simulink model "Batter_Model_01"  (R2013a)
settings: Solver=ode45  StartTime=0.0  StopTime=10.0  RelTol=1e-3
settings Model: Creator=hlopez5  LastModifiedBy=hlopez5

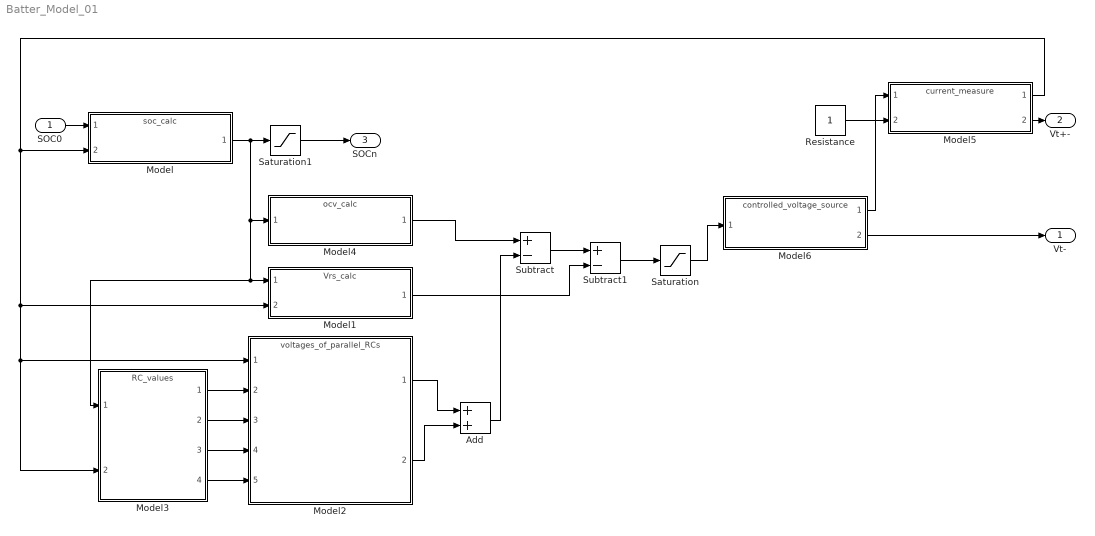
== system Batter_Model_01 ==
  SOC0 : Inport
  Add : Sum
  Model : ModelReference  ModelNameDialog=soc_calc.mdl  SimulationMode=Normal  ModelReferenceVersion=1.1  CopyOfModelName=soc_calc.mdl  DefaultDataLogging=on
  Model1 : ModelReference  ModelNameDialog=Vrs_calc.mdl  SimulationMode=Normal  ModelReferenceVersion=1.1  CopyOfModelName=Vrs_calc.mdl  DefaultDataLogging=on
  Model2 : ModelReference  ModelNameDialog=voltages_of_parallel_RCs.mdl  SimulationMode=Normal  ModelReferenceVersion=1.3  CopyOfModelName=voltages_of_parallel_RCs.mdl  DefaultDataLogging=on
  Model3 : ModelReference  ModelNameDialog=RC_values.mdl  SimulationMode=Normal  ModelReferenceVersion=1.3  CopyOfModelName=RC_values.mdl  DefaultDataLogging=on
  Model4 : ModelReference  ModelNameDialog=ocv_calc.mdl  SimulationMode=Normal  ModelReferenceVersion=1.1  CopyOfModelName=ocv_calc.mdl  DefaultDataLogging=on
  Model5 : ModelReference  ModelNameDialog=current_measure.mdl  SimulationMode=Normal  ModelReferenceVersion=1.3  CopyOfModelName=current_measure.mdl  DefaultDataLogging=on
  Model6 : ModelReference  ModelNameDialog=controlled_voltage_source.mdl  SimulationMode=Normal  ModelReferenceVersion=1.3  CopyOfModelName=controlled_voltage_source.mdl  DefaultDataLogging=on
  Resistance : Constant
  Saturation : Saturate
  Saturation1 : Saturate
  Subtract : Sum  Inputs=+-
  Subtract1 : Sum  Inputs=+-
  Vt- : Outport
  Vt+- : Outport  Port=2
  SOCn : Outport  Port=3
  wires:
  Model3/1 -> Model2/2
  Model3/2 -> Model2/3
  Model3/3 -> Model2/4
  Model3/4 -> Model2/5
  Model2/1 -> Add/1
  Model2/2 -> Add/2
  Model4/1 -> Subtract/1
  Add/1 -> Subtract/2
  Subtract/1 -> Subtract1/1
  Model1/1 -> Subtract1/2
  Subtract1/1 -> Saturation/1
  SOC0/1 -> Model/1
  Model/1 -> Model3/1, Model1/1, Model4/1, Saturation1/1
  Saturation1/1 -> SOCn/1
  Model5/1 -> Model3/2, Model2/1, Model1/2, Model/2
  Model5/2 -> Vt+-/1
  Saturation/1 -> Model6/1
  Model6/1 -> Model5/1
  Model6/2 -> Vt-/1
  Resistance/1 -> Model5/2
